simulink model "GG1Workstation_RandomCalendarTimeUntilPreempFailure"  (R2014a)
settings: Solver=ode45  SolverMode=SingleTasking  StartTime=0.0  StopTime=10000000  RelTol=1e-3
undefined symbols (not defined in the file or in its folder): se_randomizeseeds
libraries: simeventslib x8, simulink x1
settings Model: Creator=gthiers3  LastModifiedBy=AnotherUser
settings OptimizationCC: BlockReduction=off  BooleanDataType=off  SimCompilerOptimization=off
settings DebuggingCC: SaveWithParameterizedLinksMsg=none  UnderspecifiedInitializationDetection=Classic  SignalResolutionControl=TryResolveAllWithWarning  SolverPrmCheckMsg=none  FrameProcessingCompatibilityMsg=error
settings HardwareCC: TargetUnknown=on
settings RTWCC: RTWCompilerOptimization=off

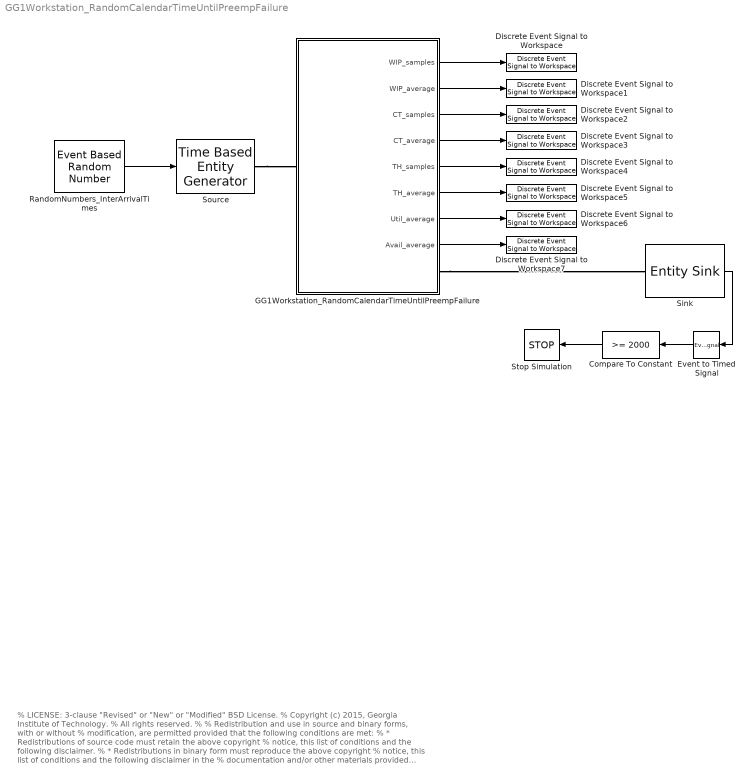
== system GG1Workstation_RandomCalendarTimeUntilPreempFailure ==
  note: % LICENSE: 3-clause "Revised" or "New" or "Modified" BSD License.
      | % Copyright (c) 2015, Georgia Institute of Technology.
      | % All rights reserved.
      | %
      | % Redistribution and use in source and binary forms, with or without
      | % modification, are permitted provided that the following conditions are met:
      | % * Redistributions of source code must retain the above copyright
      | % notice, this list of conditions and the following disclaimer.
      | % * Redistributions in binary form must reproduce the above copyright
      | % notice, this list of conditions and the following disclaimer in the
      | % documentation and/or other materials provided with the distribution.
      | % * Neither the name of the Georgia Institute of Technology nor the
      | % names of its contributors may be used to endorse or promote products
      | % derived from this software without specific prior written permission.
      | %
      | % THIS SOFTWARE IS PROVIDED BY THE COPYRIGHT HOLDERS AND CONTRIBUTORS "AS IS" AND
      | % ANY EXPRESS OR IMPLIED WARRANTIES, INCLUDING, BUT NOT LIMITED TO, THE IMPLIED
      | % WARRANTIES OF MERCHANTABILITY AND FITNESS FOR A PARTICULAR PURPOSE ARE
      | % DISCLAIMED. IN NO EVENT SHALL THE GEORGIA INSTITUTE OF TECHNOLOGY BE LIABLE FOR
      | % ANY DIRECT, INDIRECT, INCIDENTAL, SPECIAL, EXEMPLARY, OR CONSEQUENTIAL DAMAGES
      | % (INCLUDING, BUT NOT LIMITED TO, PROCUREMENT OF SUBSTITUTE GOODS OR SERVICES;
      | % LOSS OF USE, DATA, OR PROFITS; OR BUSINESS INTERRUPTION) HOWEVER CAUSED AND
      | % ON ANY THEORY OF LIABILITY, WHETHER IN CONTRACT, STRICT LIABILITY, OR TORT
      | % (INCLUDING NEGLIGENCE OR OTHERWISE) ARISING IN ANY WAY OUT OF THE USE OF THIS
      | % SOFTWARE, EVEN IF ADVISED OF THE POSSIBILITY OF SUCH DAMAGE.
  Compare To Constant : simulink/Logic and Bit Operations/Compare To Constant  relop=>=  const=2000  OutDataTypeStr=boolean
  Discrete Event Signal to Workspace : simeventslib/SimEvents Sinks/Discrete Event Signal to Workspace  VariableName=WIP_samples  SaveFormat=Structure With Time  isMonitorOnly=off  isRecordIC=off
  Discrete Event Signal to Workspace1 : simeventslib/SimEvents Sinks/Discrete Event Signal to Workspace  VariableName=WIP_average  SaveFormat=Structure With Time  isMonitorOnly=off  isRecordIC=off
  Discrete Event Signal to Workspace2 : simeventslib/SimEvents Sinks/Discrete Event Signal to Workspace  VariableName=CT_samples  SaveFormat=Structure With Time  isMonitorOnly=off  isRecordIC=off
  Discrete Event Signal to Workspace3 : simeventslib/SimEvents Sinks/Discrete Event Signal to Workspace  VariableName=CT_average  SaveFormat=Structure With Time  isMonitorOnly=off  isRecordIC=off
  Discrete Event Signal to Workspace4 : simeventslib/SimEvents Sinks/Discrete Event Signal to Workspace  VariableName=TH_samples  SaveFormat=Structure With Time  isMonitorOnly=off  isRecordIC=off
  Discrete Event Signal to Workspace5 : simeventslib/SimEvents Sinks/Discrete Event Signal to Workspace  VariableName=TH_average  SaveFormat=Structure With Time  isMonitorOnly=off  isRecordIC=off
  Discrete Event Signal to Workspace6 : simeventslib/SimEvents Sinks/Discrete Event Signal to Workspace  VariableName=Util_average  SaveFormat=Structure With Time  isMonitorOnly=off  isRecordIC=off
  Discrete Event Signal to Workspace7 : simeventslib/SimEvents Sinks/Discrete Event Signal to Workspace  VariableName=Avail_average  SaveFormat=Structure With Time  isMonitorOnly=off  isRecordIC=off
  Event to Timed Signal : EventToTimedSignal
  GG1Workstation_RandomCalendarTimeUntilPreempFailure : Subsystem  InitFcn=se_randomizeseeds(gcs, 'Mode', 'All')
      settings: CopyFcn=set_param(gcb, 'LinkStatus', 'none');
  RandomNumbers_InterArrivalTimes : EventBasedRandomNumber  meanExp=100  scaleGam=10  meanNorm=100  stdNorm=eps  Seed=6669
  Sink : EntitySink  StatNumberArrived=on
  Source : TimeBasedEntityGenerator  GenerateEntitiesUpon=Intergeneration time from port t
  Stop Simulation : Stop
  wires:
  RandomNumbers_InterArrivalTimes/1 -> Source/1
  GG1Workstation_RandomCalendarTimeUntilPreempFailure/1(WIP_samples) -> Discrete Event Signal to Workspace/1
  GG1Workstation_RandomCalendarTimeUntilPreempFailure/2(WIP_average) -> Discrete Event Signal to Workspace1/1
  GG1Workstation_RandomCalendarTimeUntilPreempFailure/3(CT_samples) -> Discrete Event Signal to Workspace2/1
  GG1Workstation_RandomCalendarTimeUntilPreempFailure/4(CT_average) -> Discrete Event Signal to Workspace3/1
  GG1Workstation_RandomCalendarTimeUntilPreempFailure/6(TH_average) -> Discrete Event Signal to Workspace5/1
  GG1Workstation_RandomCalendarTimeUntilPreempFailure/5(TH_samples) -> Discrete Event Signal to Workspace4/1
  GG1Workstation_RandomCalendarTimeUntilPreempFailure/7(Util_average) -> Discrete Event Signal to Workspace6/1
  GG1Workstation_RandomCalendarTimeUntilPreempFailure/8(Avail_average) -> Discrete Event Signal to Workspace7/1
  Event to Timed Signal/1 -> Compare To Constant/1
  Compare To Constant/1 -> Stop Simulation/1
  Sink/1 -> Event to Timed Signal/1
  connections:
  Source/RConn1 -- GG1Workstation_RandomCalendarTimeUntilPreempFailure/LConn1
  GG1Workstation_RandomCalendarTimeUntilPreempFailure/RConn1 -- Sink/LConn1

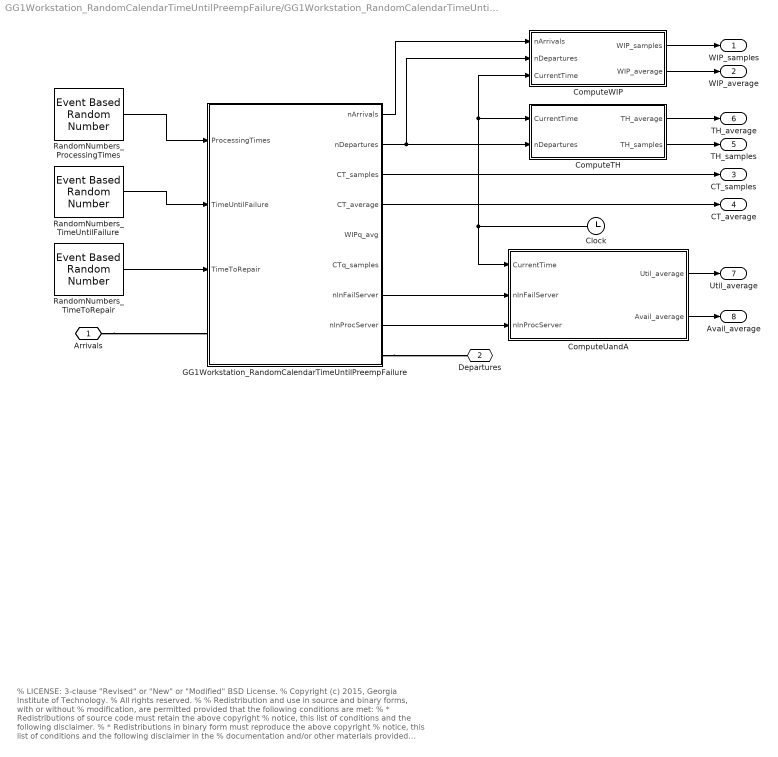
== system GG1Workstation_RandomCalendarTimeUntilPreempFailure/GG1Workstation_RandomCalendarTimeUntilPreempFailure ==
  note: % LICENSE: 3-clause "Revised" or "New" or "Modified" BSD License.
      | % Copyright (c) 2015, Georgia Institute of Technology.
      | % All rights reserved.
      | %
      | % Redistribution and use in source and binary forms, with or without
      | % modification, are permitted provided that the following conditions are met:
      | % * Redistributions of source code must retain the above copyright
      | % notice, this list of conditions and the following disclaimer.
      | % * Redistributions in binary form must reproduce the above copyright
      | % notice, this list of conditions and the following disclaimer in the
      | % documentation and/or other materials provided with the distribution.
      | % * Neither the name of the Georgia Institute of Technology nor the
      | % names of its contributors may be used to endorse or promote products
      | % derived from this software without specific prior written permission.
      | %
      | % THIS SOFTWARE IS PROVIDED BY THE COPYRIGHT HOLDERS AND CONTRIBUTORS "AS IS" AND
      | % ANY EXPRESS OR IMPLIED WARRANTIES, INCLUDING, BUT NOT LIMITED TO, THE IMPLIED
      | % WARRANTIES OF MERCHANTABILITY AND FITNESS FOR A PARTICULAR PURPOSE ARE
      | % DISCLAIMED. IN NO EVENT SHALL THE GEORGIA INSTITUTE OF TECHNOLOGY BE LIABLE FOR
      | % ANY DIRECT, INDIRECT, INCIDENTAL, SPECIAL, EXEMPLARY, OR CONSEQUENTIAL DAMAGES
      | % (INCLUDING, BUT NOT LIMITED TO, PROCUREMENT OF SUBSTITUTE GOODS OR SERVICES;
      | % LOSS OF USE, DATA, OR PROFITS; OR BUSINESS INTERRUPTION) HOWEVER CAUSED AND
      | % ON ANY THEORY OF LIABILITY, WHETHER IN CONTRACT, STRICT LIABILITY, OR TORT
      | % (INCLUDING NEGLIGENCE OR OTHERWISE) ARISING IN ANY WAY OUT OF THE USE OF THIS
      | % SOFTWARE, EVEN IF ADVISED OF THE POSSIBILITY OF SUCH DAMAGE.
  Clock : Clock
  ComputeTH : Subsystem
  ComputeUandA : Subsystem
  ComputeWIP : Subsystem
  GG1Workstation_RandomCalendarTimeUntilPreempFailure : Subsystem  mask{Capacity=Inf}
      mask prompts: Capacity "Queue Capacity"
      mask TypeOptions Capacity: FIFOQueue/Capacity
      mask DialogControl DescTextVar Prompt: GG1 Workstation, with random time intervals until preemptive failure and random repair times.  Timing is consistent with Hopp & Spearman’s model, in that the time-until-failure clock stops during repair.
  RandomNumbers_ProcessingTimes : EventBasedRandomNumber  meanExp=80  minUnif=40  maxUnif=40  pOneBern=40  pSuccessBino=40  numTrialBino=40  minTri=40  maxTri=40  modeTri=40  thresholdGam=40  scaleGam=40  shapeGam=40  meanNorm=50  stdNorm=eps  pSuccessGeo=40  meanPoiss=40  thresholdLogn=40  scaleLogn=40  shapeLogn=40  thresholdLogl=40  scaleLogl=40  minBeta=40  maxBeta=40  shape1Beta=40  shape2Beta=40  minUnid=40  maxUnid=40  numValueUnid=40  thresholdWbl=40  scaleWbl=40  shapeWbl=40  valueVecCont=40  cdfVecCont=40  valueVecDisc=40  probVecDisc=40  Seed=62554
  RandomNumbers_TimeToRepair : EventBasedRandomNumber  meanExp=400  minUnif=40  maxUnif=40  pOneBern=40  pSuccessBino=40  numTrialBino=40  minTri=38  maxTri=38  modeTri=38  scaleGam=20  meanNorm=400  stdNorm=eps  pSuccessGeo=40  meanPoiss=40  thresholdLogn=40  scaleLogn=40  shapeLogn=40  thresholdLogl=40  scaleLogl=40  minBeta=40  maxBeta=40  shape1Beta=40  shape2Beta=40  minUnid=40  maxUnid=40  numValueUnid=40  thresholdWbl=40  scaleWbl=40  shapeWbl=40  valueVecCont=40  cdfVecCont=40  probVecDisc=[0 1]  Seed=235
  RandomNumbers_TimeUntilFailure : EventBasedRandomNumber  meanExp=2500  minUnif=40  maxUnif=40  pOneBern=40  pSuccessBino=40  numTrialBino=40  minTri=114  maxTri=114  modeTri=114  scaleGam=166.6667  shapeGam=0.72  meanNorm=2000  stdNorm=eps  pSuccessGeo=40  meanPoiss=40  thresholdLogn=40  scaleLogn=40  shapeLogn=40  thresholdLogl=40  scaleLogl=40  minBeta=40  maxBeta=40  shape1Beta=40  shape2Beta=40  minUnid=40  maxUnid=40  numValueUnid=40  thresholdWbl=40  scaleWbl=40  shapeWbl=40  valueVecCont=40  cdfVecCont=40  valueVecDisc=40  probVecDisc=40  Seed=3452
  Arrivals : PMIOPort  Port=1  Side=Left
  Departures : PMIOPort  Port=2  Side=Right
  WIP_samples : Outport
  WIP_average : Outport  Port=2
  CT_samples : Outport  Port=3
  CT_average : Outport  Port=4
  TH_samples : Outport  Port=5
  TH_average : Outport  Port=6
  Util_average : Outport  Port=7
  Avail_average : Outport  Port=8
  wires:
  RandomNumbers_ProcessingTimes/1 -> GG1Workstation_RandomCalendarTimeUntilPreempFailure/1(ProcessingTimes)
  GG1Workstation_RandomCalendarTimeUntilPreempFailure/2(nDepartures) -> ComputeTH/2(nDepartures), ComputeWIP/2(nDepartures)
  GG1Workstation_RandomCalendarTimeUntilPreempFailure/3(CT_samples) -> CT_samples/1
  GG1Workstation_RandomCalendarTimeUntilPreempFailure/4(CT_average) -> CT_average/1
  ComputeWIP/1(WIP_samples) -> WIP_samples/1
  ComputeWIP/2(WIP_average) -> WIP_average/1
  GG1Workstation_RandomCalendarTimeUntilPreempFailure/1(nArrivals) -> ComputeWIP/1(nArrivals)
  Clock/1 -> ComputeUandA/1(CurrentTime), ComputeTH/1(CurrentTime), ComputeWIP/3(CurrentTime)
  ComputeTH/1(TH_average) -> TH_average/1
  ComputeTH/2(TH_samples) -> TH_samples/1
  RandomNumbers_TimeUntilFailure/1 -> GG1Workstation_RandomCalendarTimeUntilPreempFailure/2(TimeUntilFailure)
  RandomNumbers_TimeToRepair/1 -> GG1Workstation_RandomCalendarTimeUntilPreempFailure/3(TimeToRepair)
  GG1Workstation_RandomCalendarTimeUntilPreempFailure/7(nInFailServer) -> ComputeUandA/2(nInFailServer)
  GG1Workstation_RandomCalendarTimeUntilPreempFailure/8(nInProcServer) -> ComputeUandA/3(nInProcServer)
  ComputeUandA/1(Util_average) -> Util_average/1
  ComputeUandA/2(Avail_average) -> Avail_average/1
  connections:
  GG1Workstation_RandomCalendarTimeUntilPreempFailure/RConn1 -- Departures/RConn1
  Arrivals/RConn1 -- GG1Workstation_RandomCalendarTimeUntilPreempFailure/LConn1

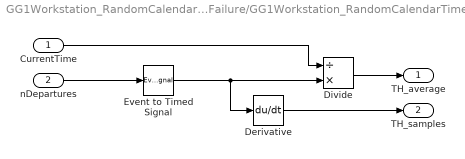
== system GG1Workstation_RandomCalendarTimeUntilPreempFailure/GG1Workstation_RandomCalendarTimeUntilPreempFailure/ComputeTH ==
  CurrentTime : Inport
  nDepartures : Inport  Port=2
  Derivative : Derivative
  Divide : Product  Inputs=/*
  Event to Timed Signal : EventToTimedSignal
  TH_average : Outport
  TH_samples : Outport  Port=2
  wires:
  CurrentTime/1 -> Divide/1
  Event to Timed Signal/1 -> Derivative/1, Divide/2
  Divide/1 -> TH_average/1
  Derivative/1 -> TH_samples/1
  nDepartures/1 -> Event to Timed Signal/1

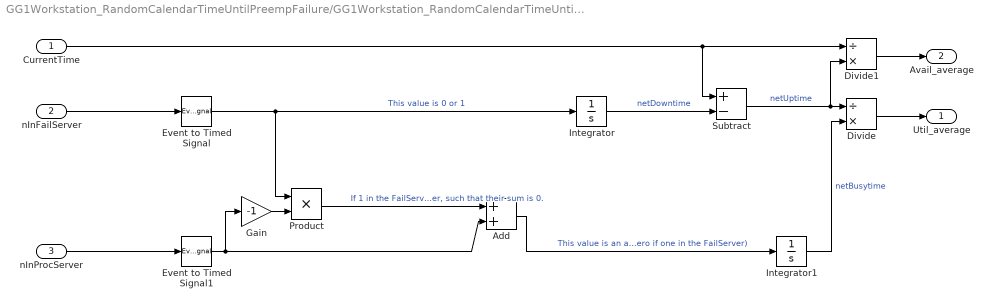
== system GG1Workstation_RandomCalendarTimeUntilPreempFailure/GG1Workstation_RandomCalendarTimeUntilPreempFailure/ComputeUandA ==
  CurrentTime : Inport
  nInFailServer : Inport  Port=2
  nInProcServer : Inport  Port=3
  Add : Sum
  Divide : Product  Inputs=/*
  Divide1 : Product  Inputs=/*
  Event to Timed Signal : EventToTimedSignal
  Event to Timed Signal1 : EventToTimedSignal
  Gain : Gain  Gain=-1
  Integrator : Integrator
  Integrator1 : Integrator
  Product : Product
  Subtract : Sum  Inputs=+-
  Util_average : Outport
  Avail_average : Outport  Port=2
  wires:
  Event to Timed Signal/1 -> Integrator/1, Product/1  "This value is 0 or 1"
  nInFailServer/1 -> Event to Timed Signal/1
  nInProcServer/1 -> Event to Timed Signal1/1
  Integrator/1 -> Subtract/2  "netDowntime"
  CurrentTime/1 -> Subtract/1, Divide1/1
  Divide/1 -> Util_average/1
  Subtract/1 -> Divide/1, Divide1/2  "netUptime"
  Integrator1/1 -> Divide/2  "netBusytime"
  Gain/1 -> Product/2
  Product/1 -> Add/1  "If 1 in the FailServer, then this value should be negative the number in the ProcServer, such that their sum is 0."
  Add/1 -> Integrator1/1  "This value is an adjusted number in the ProcServer (zero if one in the FailServer)"
  Event to Timed Signal1/1 -> Add/2, Gain/1
  Divide1/1 -> Avail_average/1

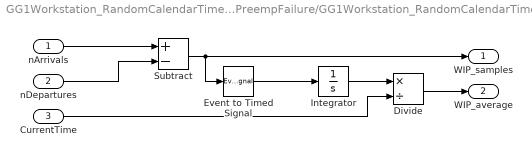
== system GG1Workstation_RandomCalendarTimeUntilPreempFailure/GG1Workstation_RandomCalendarTimeUntilPreempFailure/ComputeWIP ==
  nArrivals : Inport
  nDepartures : Inport  Port=2
  CurrentTime : Inport  Port=3
  Divide : Product  Inputs=*/
  Event to Timed Signal : EventToTimedSignal
  Integrator : Integrator
  Subtract : Sum  Inputs=+-
  WIP_samples : Outport
  WIP_average : Outport  Port=2
  wires:
  Subtract/1 -> WIP_samples/1, Event to Timed Signal/1
  Event to Timed Signal/1 -> Integrator/1
  Divide/1 -> WIP_average/1
  Integrator/1 -> Divide/1
  nArrivals/1 -> Subtract/1
  nDepartures/1 -> Subtract/2
  CurrentTime/1 -> Divide/2

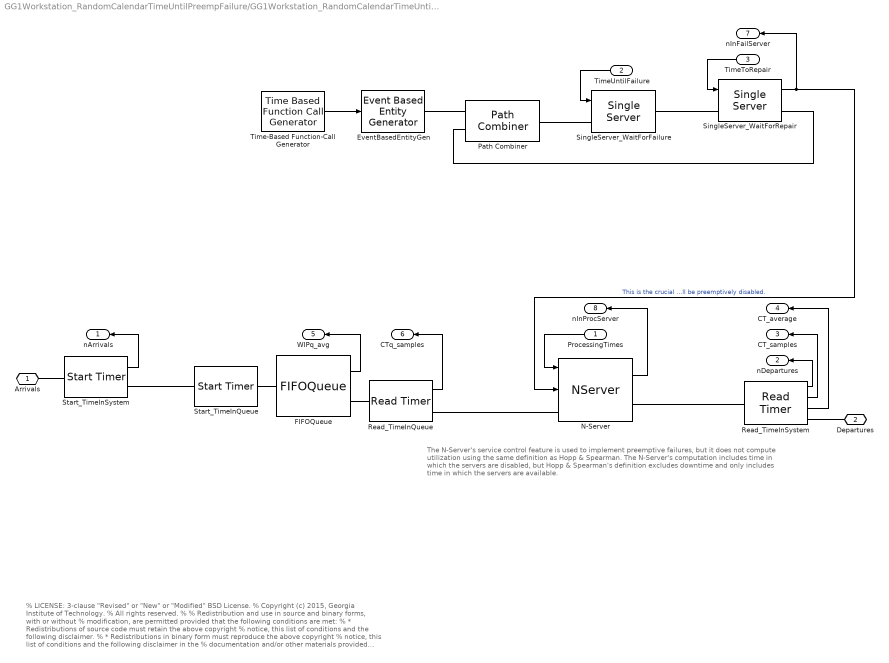
== system GG1Workstation_RandomCalendarTimeUntilPreempFailure/GG1Workstation_RandomCalendarTimeUntilPreempFailure/GG1Workstation_RandomCalendarTimeUntilPreempFailure ==
  note: The N-Server's service control feature is used to implement preemptive failures,
      | but it does not compute utilization using the same definition as Hopp & Spearman.
      | The N-Server's computation includes time in which the servers are disabled, but
      | Hopp & Spearman's definition excludes downtime and only includes time in which
      | the servers are available.
  note: % LICENSE: 3-clause "Revised" or "New" or "Modified" BSD License.
      | % Copyright (c) 2015, Georgia Institute of Technology.
      | % All rights reserved.
      | %
      | % Redistribution and use in source and binary forms, with or without
      | % modification, are permitted provided that the following conditions are met:
      | % * Redistributions of source code must retain the above copyright
      | % notice, this list of conditions and the following disclaimer.
      | % * Redistributions in binary form must reproduce the above copyright
      | % notice, this list of conditions and the following disclaimer in the
      | % documentation and/or other materials provided with the distribution.
      | % * Neither the name of the Georgia Institute of Technology nor the
      | % names of its contributors may be used to endorse or promote products
      | % derived from this software without specific prior written permission.
      | %
      | % THIS SOFTWARE IS PROVIDED BY THE COPYRIGHT HOLDERS AND CONTRIBUTORS "AS IS" AND
      | % ANY EXPRESS OR IMPLIED WARRANTIES, INCLUDING, BUT NOT LIMITED TO, THE IMPLIED
      | % WARRANTIES OF MERCHANTABILITY AND FITNESS FOR A PARTICULAR PURPOSE ARE
      | % DISCLAIMED. IN NO EVENT SHALL THE GEORGIA INSTITUTE OF TECHNOLOGY BE LIABLE FOR
      | % ANY DIRECT, INDIRECT, INCIDENTAL, SPECIAL, EXEMPLARY, OR CONSEQUENTIAL DAMAGES
      | % (INCLUDING, BUT NOT LIMITED TO, PROCUREMENT OF SUBSTITUTE GOODS OR SERVICES;
      | % LOSS OF USE, DATA, OR PROFITS; OR BUSINESS INTERRUPTION) HOWEVER CAUSED AND
      | % ON ANY THEORY OF LIABILITY, WHETHER IN CONTRACT, STRICT LIABILITY, OR TORT
      | % (INCLUDING NEGLIGENCE OR OTHERWISE) ARISING IN ANY WAY OUT OF THE USE OF THIS
      | % SOFTWARE, EVEN IF ADVISED OF THE POSSIBILITY OF SUCH DAMAGE.
  ProcessingTimes : Inport
  TimeUntilFailure : Inport  Port=2
  TimeToRepair : Inport  Port=3
  EventBasedEntityGen : EventBasedEntityGenerator  GenerateEntitiesUpon=Function call from port fcn
  FIFOQueue : FIFOQueue  Capacity=Capacity  StatAverageQueueLength=on
      settings: OutputPortMap=o3
  N-Server : NServer  NumberOfServers=1  ServiceTimeFrom=Signal port t  ServiceTime=0  AttributeName=ProcTime  AllowServiceControl=on  BlockWhileSignalOn=on  StatNumberInBlock=on
      settings: InputPortMap=u0,u1  OutputPortMap=o1
  Path Combiner : PathCombiner  NumberInputPorts=2
  Read_TimeInQueue : ReadTimer  TimerTag=TimeInQueue  StatTimeElapsed=on
      settings: OutputPortMap=o2
  Read_TimeInSystem : ReadTimer  TimerTag=TimeInSystem  StatNumberDeparted=on  StatTimeElapsed=on  StatAverageTimeElapsed=on
      settings: OutputPortMap=o0,o2,o3
  SingleServer_WaitForFailure : SingleServer  ServiceTimeFrom=Signal port t  AttributeName=TimeUntilFailure
  SingleServer_WaitForRepair : SingleServer  ServiceTimeFrom=Signal port t  AttributeName=TimeToRepair  StatNumberInBlock=on
      settings: OutputPortMap=o1
  Start_TimeInQueue : StartTimer  TimerTag=TimeInQueue  TimerStartedOption=Restart
  Start_TimeInSystem : StartTimer  TimerTag=TimeInSystem  TimerStartedOption=Restart  StatNumberDeparted=on
  Time-Based Function-Call Generator : TimeBasedFunctionCallGenerator  EventGenerationMode=Only at simulation start
  Arrivals : PMIOPort  Port=1  Side=Left
  Departures : PMIOPort  Port=2  Side=Right
  nArrivals : Outport
  nDepartures : Outport  Port=2
  CT_samples : Outport  Port=3
  CT_average : Outport  Port=4
  WIPq_avg : Outport  Port=5
  CTq_samples : Outport  Port=6
  nInFailServer : Outport  Port=7
  nInProcServer : Outport  Port=8
  wires:
  Read_TimeInSystem/2 -> CT_samples/1
  Read_TimeInQueue/1 -> CTq_samples/1
  FIFOQueue/1 -> WIPq_avg/1
  Start_TimeInSystem/1 -> nArrivals/1
  Read_TimeInSystem/1 -> nDepartures/1
  Read_TimeInSystem/3 -> CT_average/1
  Time-Based Function-Call Generator/1 -> EventBasedEntityGen/1
  SingleServer_WaitForRepair/1 -> N-Server/2, nInFailServer/1  "This is the crucial blocking signal. When > 0, the N-Server will be preemptively disabled."
  ProcessingTimes/1 -> N-Server/1
  N-Server/1 -> nInProcServer/1
  TimeToRepair/1 -> SingleServer_WaitForRepair/1
  TimeUntilFailure/1 -> SingleServer_WaitForFailure/1
  connections:
  FIFOQueue/RConn1 -- Read_TimeInQueue/LConn1
  Start_TimeInSystem/RConn1 -- Start_TimeInQueue/LConn1
  Read_TimeInSystem/RConn1 -- Departures/RConn1
  Start_TimeInQueue/RConn1 -- FIFOQueue/LConn1
  SingleServer_WaitForRepair/LConn1 -- SingleServer_WaitForFailure/RConn1
  EventBasedEntityGen/RConn1 -- Path Combiner/LConn1
  Path Combiner/LConn2 -- SingleServer_WaitForRepair/RConn1
  Read_TimeInQueue/RConn1 -- N-Server/LConn1
  Arrivals/RConn1 -- Start_TimeInSystem/LConn1
  N-Server/RConn1 -- Read_TimeInSystem/LConn1
  Path Combiner/RConn1 -- SingleServer_WaitForFailure/LConn1
